simulink library "Labor02"  (R2018b)
settings: Solver=VariableStepAuto  StartTime=0.0  StopTime=10.0  RelTol=1e-3
values from neighbouring files (symbols this model uses):
  A = 0.01266    [var.m]    (also in var.mat)
  G = 1200    [var.m]    (also in var.mat = 1000)
  G_n = 1000    [var.m]    (also in var.mat)
  I_0 = 2.8e-9    (= 2.8e-09)    [var.m]    (also in var.mat)
  J_sc = 343    [var.m]    (also in var.mat)
  k = 1.38064852*10^-23    (= 1.38064852e-23)    [var.m]    (also in var.mat)
  m = 1    [var.m]    (also in var.mat)
  q = 1.602176565*10^-19    (= 1.602176565e-19)    [var.m]    (also in var.mat)
  R_s = 1e-6    (= 1e-06)    [var.m]    (also in var.mat)
  R_sh = 1000    [var.m]    (also in var.mat)
  T = 50 + 273.15    (= 323.15)    [var.m]    (also in var.mat = 300)
  V = 0.5    [var.m]    (also in var.mat)
  Vt = 25.85e-3    (= 0.02585)    [var.m]    (also in var.mat)
settings Model: Creator=heerdavi18  LastModifiedBy=diktux

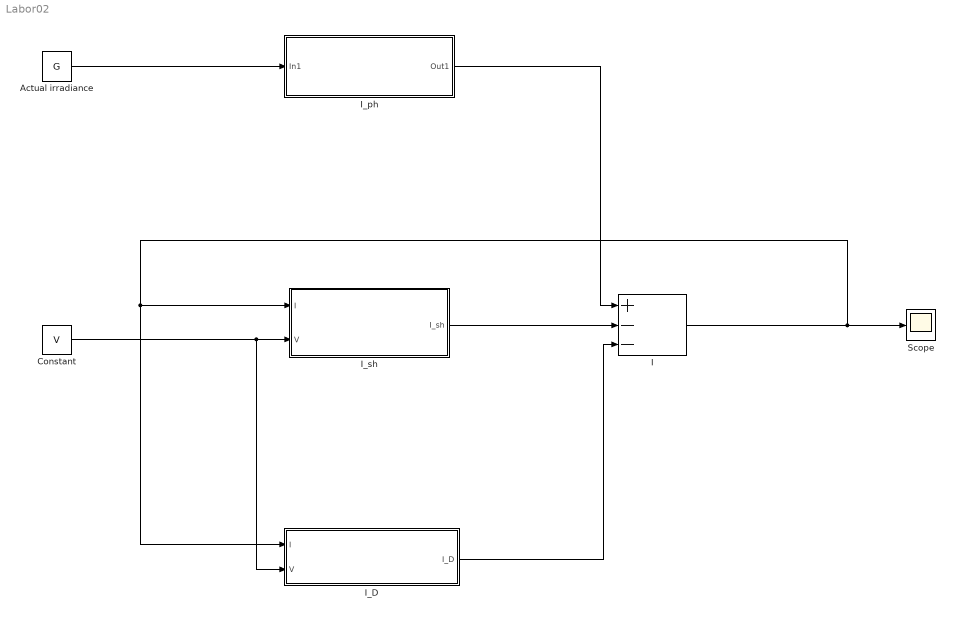
== system Labor02 ==
  Actual irradiance : Constant  Value=G
  Constant : Constant  Value=V
  I : Sum  Inputs=+--
  I_D : Subsystem
  "I_ph " : Subsystem
  I_sh : Subsystem
  Scope : Scope
  wires:
  Actual irradiance/1 -> "I_ph "/1(In1)
  "I_ph "/1(Out1) -> I/1
  I/1 -> I_D/1(I), I_sh/1(I), Scope/1
  Constant/1 -> I_D/2(V), I_sh/2(V)
  I_sh/1(I_sh) -> I/2
  I_D/1(I_D) -> I/3

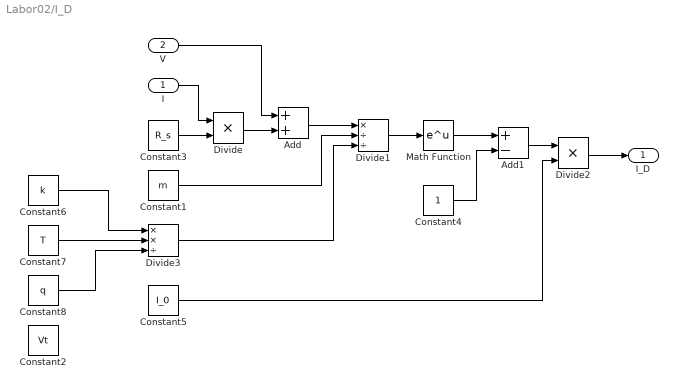
== system Labor02/I_D ==
  I : Inport
  V : Inport  Port=2
  Add : Sum
  Add1 : Sum  Inputs=+-
  Constant1 : Constant  Value=m
  Constant2 : Constant  Value=Vt
  Constant3 : Constant  Value=R_s
  Constant4 : Constant
  Constant5 : Constant  Value=I_0
  Constant6 : Constant  Value=k
  Constant7 : Constant  Value=T
  Constant8 : Constant  Value=q
  Divide : Product  Inputs=**
  Divide1 : Product  Inputs=*//
  Divide2 : Product  Inputs=**
  Divide3 : Product  Inputs=**/
  Math Function : Math  SaturateOnIntegerOverflow=on
  I_D : Outport
  wires:
  Constant4/1 -> Add1/2
  Constant3/1 -> Divide/2
  Divide1/1 -> Math Function/1
  Add/1 -> Divide1/1
  Divide/1 -> Add/2
  Constant1/1 -> Divide1/2
  Math Function/1 -> Add1/1
  Add1/1 -> Divide2/1
  Constant5/1 -> Divide2/2
  V/1 -> Add/1
  Divide2/1 -> I_D/1
  I/1 -> Divide/1
  Constant8/1 -> Divide3/3
  Constant7/1 -> Divide3/2
  Constant6/1 -> Divide3/1
  Divide3/1 -> Divide1/3

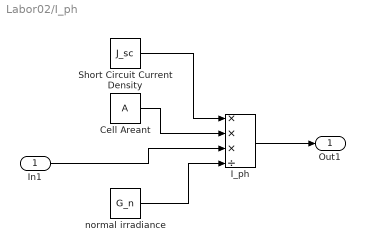
== system Labor02/I_ph  ==
  In1 : Inport
  Cell Areant : Constant  Value=A
  I_ph : Product  Inputs=***/
  Short Circuit Current Density : Constant  Value=J_sc
  normal irradiance : Constant  Value=G_n
  Out1 : Outport
  wires:
  Cell Areant/1 -> I_ph/2
  I_ph/1 -> Out1/1
  Short Circuit Current Density/1 -> I_ph/1
  In1/1 -> I_ph/3
  normal irradiance/1 -> I_ph/4

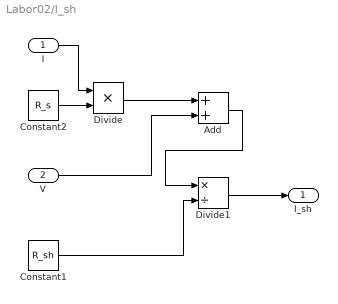
== system Labor02/I_sh ==
  I : Inport
  V : Inport  Port=2
  Add : Sum
  Constant1 : Constant  Value=R_sh
  Constant2 : Constant  Value=R_s
  Divide : Product  Inputs=**
  Divide1 : Product  Inputs=*/
  I_sh : Outport
  wires:
  Constant2/1 -> Divide/2
  Constant1/1 -> Divide1/2
  I/1 -> Divide/1
  V/1 -> Add/2
  Divide/1 -> Add/1
  Add/1 -> Divide1/1
  Divide1/1 -> I_sh/1
